simulink model "ALU_04_SS"  (R2022a)
settings: Solver=VariableStepAuto  StartTime=0.0  StopTime=10.0  RelTol=1e-3
undefined symbols (not defined in the file or in its folder): xc7z010iclg225
libraries: hdlBasic x1537, vmcUtilities x1
(part 8 of 8)

== system ALU_04_SS/ALU_64_BITS/ALU_63 ==
  CARRY_IN (1 BIT) : Inport
  OP (2 BIT) : Inport  Port=2
  A_INVERT (1 BIT) : Inport  Port=3
  A_INPUT (1 BIT) : Inport  Port=4
  B_INVERT (1 BIT) : Inport  Port=5
  B_INPUT (1 BIT) : Inport  Port=6
  Inverter{1..3,8..9} (5 alike) : hdlBasic/Inverter  en=off  latency=0  XmcBlockStatus=1  maskContainerNames=group2  block_type=inv  block_config=sysgen:Inverter_config
  Logical{,1..3} (4 alike) : hdlBasic/Logical  logical_function=AND  inputs=2  en=off  latency=0  precision=Full  arith_type=Unsigned  n_bits=16  bin_pt=0  align_bp=on  overflow=[]  quantization=[]  XmcBlockStatus=1  maskContainerNames=tabcontainer1  block_type=logical  block_config=sysgen:Logical_config
  Logical{4..6,9} (4 alike) : hdlBasic/Logical  logical_function=AND  inputs=3  en=off  latency=0  precision=Full  arith_type=Unsigned  n_bits=16  bin_pt=0  align_bp=on  overflow=[]  quantization=[]  XmcBlockStatus=1  maskContainerNames=tabcontainer1  block_type=logical  block_config=sysgen:Logical_config
  Logical7 : hdlBasic/Logical  logical_function=OR  inputs=2  en=off  latency=0  precision=Full  arith_type=Unsigned  n_bits=16  bin_pt=0  align_bp=on  overflow=[]  quantization=[]  XmcBlockStatus=1  maskContainerNames=tabcontainer1  block_type=logical  block_config=sysgen:Logical_config
  Logical8 : hdlBasic/Logical  logical_function=XOR  inputs=2  en=off  latency=0  precision=Full  arith_type=Unsigned  n_bits=16  bin_pt=0  align_bp=on  overflow=[]  quantization=[]  XmcBlockStatus=1  maskContainerNames=tabcontainer1  block_type=logical  block_config=sysgen:Logical_config
  Mux : hdlBasic/Mux  inputs=4  en=off  latency=0  precision=Full  arith_type=Unsigned  n_bits=16  bin_pt=14  quantization=Truncate  overflow=Wrap  XmcBlockStatus=1  maskContainerNames=tabcontainer1  block_type=mux  block_config=sysgen:Mux_config
  Mux1 : hdlBasic/Mux  inputs=2  en=off  latency=0  precision=Full  arith_type=Unsigned  n_bits=16  bin_pt=14  quantization=Truncate  overflow=Wrap  XmcBlockStatus=1  maskContainerNames=tabcontainer1  block_type=mux  block_config=sysgen:Mux_config
  Mux2 : hdlBasic/Mux  inputs=2  en=off  latency=0  precision=Full  arith_type=Unsigned  n_bits=16  bin_pt=14  quantization=Truncate  overflow=Wrap  XmcBlockStatus=1  maskContainerNames=tabcontainer1  block_type=mux  block_config=sysgen:Mux_config
  Sum : hdlBasic/Logical  logical_function=OR  inputs=4  en=off  latency=0  precision=Full  arith_type=Unsigned  n_bits=16  bin_pt=0  align_bp=on  overflow=[]  quantization=[]  XmcBlockStatus=1  maskContainerNames=tabcontainer1  block_type=logical  block_config=sysgen:Logical_config
  c_out : hdlBasic/Logical  logical_function=OR  inputs=3  en=off  latency=0  precision=Full  arith_type=Unsigned  n_bits=16  bin_pt=0  align_bp=on  overflow=[]  quantization=[]  XmcBlockStatus=1  maskContainerNames=tabcontainer1  block_type=logical  block_config=sysgen:Logical_config
  ALU_OUT (1 BIT) : Outport
  CARRY_OUT (1 BIT) : Outport  Port=2
  wires:
  Logical2/1 -> c_out/3
  A_INVERT (1 BIT)/1 -> Mux1/1
  c_out/1 -> CARRY_OUT (1 BIT)/1
  Sum/1 -> Mux/4
  CARRY_IN (1 BIT)/1 -> Inverter1/1, Logical5/1, Logical4/1, Logical1/1, Logical/1
  Mux2/1 -> Logical5/3, Logical6/3, Logical1/2, Logical2/2, Inverter9/1, Logical8/2, Logical3/2, Logical7/2
  B_INPUT (1 BIT)/1 -> Inverter3/1, Mux2/2
  Mux/1 -> ALU_OUT (1 BIT)/1
  Logical/1 -> c_out/1
  B_INVERT (1 BIT)/1 -> Mux2/1
  Logical6/1 -> Sum/3
  Mux1/1 -> Logical8/1, Logical7/1, Logical3/1, Inverter8/1, Logical5/2, Logical/2, Logical2/1, Logical9/2
  Logical5/1 -> Sum/4
  OP (2 BIT)/1 -> Mux/1
  Logical9/1 -> Sum/2
  Inverter1/1 -> Logical6/1, Logical9/1
  Inverter3/1 -> Mux2/3
  Inverter9/1 -> Logical9/3, Logical4/3
  A_INPUT (1 BIT)/1 -> Mux1/2, Inverter2/1
  Inverter2/1 -> Mux1/3
  Logical4/1 -> Sum/1
  Inverter8/1 -> Logical6/2, Logical4/2
  Logical3/1 -> Mux/2
  Logical7/1 -> Mux/3
  Logical1/1 -> c_out/2
  Logical8/1 -> Mux/5

== system ALU_04_SS/ALU_64_BITS/ALU_7 ==
  CARRY_IN (1 BIT) : Inport
  OP (2 BIT) : Inport  Port=2
  A_INVERT (1 BIT) : Inport  Port=3
  A_INPUT (1 BIT) : Inport  Port=4
  B_INVERT (1 BIT) : Inport  Port=5
  B_INPUT (1 BIT) : Inport  Port=6
  Inverter{1..3,8..9} (5 alike) : hdlBasic/Inverter  en=off  latency=0  XmcBlockStatus=1  maskContainerNames=group2  block_type=inv  block_config=sysgen:Inverter_config
  Logical{,1..3} (4 alike) : hdlBasic/Logical  logical_function=AND  inputs=2  en=off  latency=0  precision=Full  arith_type=Unsigned  n_bits=16  bin_pt=0  align_bp=on  overflow=[]  quantization=[]  XmcBlockStatus=1  maskContainerNames=tabcontainer1  block_type=logical  block_config=sysgen:Logical_config
  Logical{4..6,9} (4 alike) : hdlBasic/Logical  logical_function=AND  inputs=3  en=off  latency=0  precision=Full  arith_type=Unsigned  n_bits=16  bin_pt=0  align_bp=on  overflow=[]  quantization=[]  XmcBlockStatus=1  maskContainerNames=tabcontainer1  block_type=logical  block_config=sysgen:Logical_config
  Logical7 : hdlBasic/Logical  logical_function=OR  inputs=2  en=off  latency=0  precision=Full  arith_type=Unsigned  n_bits=16  bin_pt=0  align_bp=on  overflow=[]  quantization=[]  XmcBlockStatus=1  maskContainerNames=tabcontainer1  block_type=logical  block_config=sysgen:Logical_config
  Logical8 : hdlBasic/Logical  logical_function=XOR  inputs=2  en=off  latency=0  precision=Full  arith_type=Unsigned  n_bits=16  bin_pt=0  align_bp=on  overflow=[]  quantization=[]  XmcBlockStatus=1  maskContainerNames=tabcontainer1  block_type=logical  block_config=sysgen:Logical_config
  Mux : hdlBasic/Mux  inputs=4  en=off  latency=0  precision=Full  arith_type=Unsigned  n_bits=16  bin_pt=14  quantization=Truncate  overflow=Wrap  XmcBlockStatus=1  maskContainerNames=tabcontainer1  block_type=mux  block_config=sysgen:Mux_config
  Mux1 : hdlBasic/Mux  inputs=2  en=off  latency=0  precision=Full  arith_type=Unsigned  n_bits=16  bin_pt=14  quantization=Truncate  overflow=Wrap  XmcBlockStatus=1  maskContainerNames=tabcontainer1  block_type=mux  block_config=sysgen:Mux_config
  Mux2 : hdlBasic/Mux  inputs=2  en=off  latency=0  precision=Full  arith_type=Unsigned  n_bits=16  bin_pt=14  quantization=Truncate  overflow=Wrap  XmcBlockStatus=1  maskContainerNames=tabcontainer1  block_type=mux  block_config=sysgen:Mux_config
  Sum : hdlBasic/Logical  logical_function=OR  inputs=4  en=off  latency=0  precision=Full  arith_type=Unsigned  n_bits=16  bin_pt=0  align_bp=on  overflow=[]  quantization=[]  XmcBlockStatus=1  maskContainerNames=tabcontainer1  block_type=logical  block_config=sysgen:Logical_config
  c_out : hdlBasic/Logical  logical_function=OR  inputs=3  en=off  latency=0  precision=Full  arith_type=Unsigned  n_bits=16  bin_pt=0  align_bp=on  overflow=[]  quantization=[]  XmcBlockStatus=1  maskContainerNames=tabcontainer1  block_type=logical  block_config=sysgen:Logical_config
  ALU_OUT (1 BIT) : Outport
  CARRY_OUT (1 BIT) : Outport  Port=2
  wires:
  Logical2/1 -> c_out/3
  A_INVERT (1 BIT)/1 -> Mux1/1
  c_out/1 -> CARRY_OUT (1 BIT)/1
  Sum/1 -> Mux/4
  CARRY_IN (1 BIT)/1 -> Inverter1/1, Logical5/1, Logical4/1, Logical1/1, Logical/1
  Mux2/1 -> Logical5/3, Logical6/3, Logical1/2, Logical2/2, Inverter9/1, Logical8/2, Logical3/2, Logical7/2
  B_INPUT (1 BIT)/1 -> Inverter3/1, Mux2/2
  Mux/1 -> ALU_OUT (1 BIT)/1
  Logical/1 -> c_out/1
  B_INVERT (1 BIT)/1 -> Mux2/1
  Logical6/1 -> Sum/3
  Mux1/1 -> Logical8/1, Logical7/1, Logical3/1, Inverter8/1, Logical5/2, Logical/2, Logical2/1, Logical9/2
  Logical5/1 -> Sum/4
  OP (2 BIT)/1 -> Mux/1
  Logical9/1 -> Sum/2
  Inverter1/1 -> Logical6/1, Logical9/1
  Inverter3/1 -> Mux2/3
  Inverter9/1 -> Logical9/3, Logical4/3
  A_INPUT (1 BIT)/1 -> Mux1/2, Inverter2/1
  Inverter2/1 -> Mux1/3
  Logical4/1 -> Sum/1
  Inverter8/1 -> Logical6/2, Logical4/2
  Logical3/1 -> Mux/2
  Logical7/1 -> Mux/3
  Logical1/1 -> c_out/2
  Logical8/1 -> Mux/5

== system ALU_04_SS/ALU_64_BITS/ALU_8 ==
  CARRY_IN (1 BIT) : Inport
  OP (2 BIT) : Inport  Port=2
  A_INVERT (1 BIT) : Inport  Port=3
  A_INPUT (1 BIT) : Inport  Port=4
  B_INVERT (1 BIT) : Inport  Port=5
  B_INPUT (1 BIT) : Inport  Port=6
  Inverter{1..3,8..9} (5 alike) : hdlBasic/Inverter  en=off  latency=0  XmcBlockStatus=1  maskContainerNames=group2  block_type=inv  block_config=sysgen:Inverter_config
  Logical{,1..3} (4 alike) : hdlBasic/Logical  logical_function=AND  inputs=2  en=off  latency=0  precision=Full  arith_type=Unsigned  n_bits=16  bin_pt=0  align_bp=on  overflow=[]  quantization=[]  XmcBlockStatus=1  maskContainerNames=tabcontainer1  block_type=logical  block_config=sysgen:Logical_config
  Logical{4..6,9} (4 alike) : hdlBasic/Logical  logical_function=AND  inputs=3  en=off  latency=0  precision=Full  arith_type=Unsigned  n_bits=16  bin_pt=0  align_bp=on  overflow=[]  quantization=[]  XmcBlockStatus=1  maskContainerNames=tabcontainer1  block_type=logical  block_config=sysgen:Logical_config
  Logical7 : hdlBasic/Logical  logical_function=OR  inputs=2  en=off  latency=0  precision=Full  arith_type=Unsigned  n_bits=16  bin_pt=0  align_bp=on  overflow=[]  quantization=[]  XmcBlockStatus=1  maskContainerNames=tabcontainer1  block_type=logical  block_config=sysgen:Logical_config
  Logical8 : hdlBasic/Logical  logical_function=XOR  inputs=2  en=off  latency=0  precision=Full  arith_type=Unsigned  n_bits=16  bin_pt=0  align_bp=on  overflow=[]  quantization=[]  XmcBlockStatus=1  maskContainerNames=tabcontainer1  block_type=logical  block_config=sysgen:Logical_config
  Mux : hdlBasic/Mux  inputs=4  en=off  latency=0  precision=Full  arith_type=Unsigned  n_bits=16  bin_pt=14  quantization=Truncate  overflow=Wrap  XmcBlockStatus=1  maskContainerNames=tabcontainer1  block_type=mux  block_config=sysgen:Mux_config
  Mux1 : hdlBasic/Mux  inputs=2  en=off  latency=0  precision=Full  arith_type=Unsigned  n_bits=16  bin_pt=14  quantization=Truncate  overflow=Wrap  XmcBlockStatus=1  maskContainerNames=tabcontainer1  block_type=mux  block_config=sysgen:Mux_config
  Mux2 : hdlBasic/Mux  inputs=2  en=off  latency=0  precision=Full  arith_type=Unsigned  n_bits=16  bin_pt=14  quantization=Truncate  overflow=Wrap  XmcBlockStatus=1  maskContainerNames=tabcontainer1  block_type=mux  block_config=sysgen:Mux_config
  Sum : hdlBasic/Logical  logical_function=OR  inputs=4  en=off  latency=0  precision=Full  arith_type=Unsigned  n_bits=16  bin_pt=0  align_bp=on  overflow=[]  quantization=[]  XmcBlockStatus=1  maskContainerNames=tabcontainer1  block_type=logical  block_config=sysgen:Logical_config
  c_out : hdlBasic/Logical  logical_function=OR  inputs=3  en=off  latency=0  precision=Full  arith_type=Unsigned  n_bits=16  bin_pt=0  align_bp=on  overflow=[]  quantization=[]  XmcBlockStatus=1  maskContainerNames=tabcontainer1  block_type=logical  block_config=sysgen:Logical_config
  ALU_OUT (1 BIT) : Outport
  CARRY_OUT (1 BIT) : Outport  Port=2
  wires:
  Logical2/1 -> c_out/3
  A_INVERT (1 BIT)/1 -> Mux1/1
  c_out/1 -> CARRY_OUT (1 BIT)/1
  Sum/1 -> Mux/4
  CARRY_IN (1 BIT)/1 -> Inverter1/1, Logical5/1, Logical4/1, Logical1/1, Logical/1
  Mux2/1 -> Logical5/3, Logical6/3, Logical1/2, Logical2/2, Inverter9/1, Logical8/2, Logical3/2, Logical7/2
  B_INPUT (1 BIT)/1 -> Inverter3/1, Mux2/2
  Mux/1 -> ALU_OUT (1 BIT)/1
  Logical/1 -> c_out/1
  B_INVERT (1 BIT)/1 -> Mux2/1
  Logical6/1 -> Sum/3
  Mux1/1 -> Logical8/1, Logical7/1, Logical3/1, Inverter8/1, Logical5/2, Logical/2, Logical2/1, Logical9/2
  Logical5/1 -> Sum/4
  OP (2 BIT)/1 -> Mux/1
  Logical9/1 -> Sum/2
  Inverter1/1 -> Logical6/1, Logical9/1
  Inverter3/1 -> Mux2/3
  Inverter9/1 -> Logical9/3, Logical4/3
  A_INPUT (1 BIT)/1 -> Mux1/2, Inverter2/1
  Inverter2/1 -> Mux1/3
  Logical4/1 -> Sum/1
  Inverter8/1 -> Logical6/2, Logical4/2
  Logical3/1 -> Mux/2
  Logical7/1 -> Mux/3
  Logical1/1 -> c_out/2
  Logical8/1 -> Mux/5

== system ALU_04_SS/ALU_64_BITS/ALU_9 ==
  CARRY_IN (1 BIT) : Inport
  OP (2 BIT) : Inport  Port=2
  A_INVERT (1 BIT) : Inport  Port=3
  A_INPUT (1 BIT) : Inport  Port=4
  B_INVERT (1 BIT) : Inport  Port=5
  B_INPUT (1 BIT) : Inport  Port=6
  Inverter{1..3,8..9} (5 alike) : hdlBasic/Inverter  en=off  latency=0  XmcBlockStatus=1  maskContainerNames=group2  block_type=inv  block_config=sysgen:Inverter_config
  Logical{,1..3} (4 alike) : hdlBasic/Logical  logical_function=AND  inputs=2  en=off  latency=0  precision=Full  arith_type=Unsigned  n_bits=16  bin_pt=0  align_bp=on  overflow=[]  quantization=[]  XmcBlockStatus=1  maskContainerNames=tabcontainer1  block_type=logical  block_config=sysgen:Logical_config
  Logical{4..6,9} (4 alike) : hdlBasic/Logical  logical_function=AND  inputs=3  en=off  latency=0  precision=Full  arith_type=Unsigned  n_bits=16  bin_pt=0  align_bp=on  overflow=[]  quantization=[]  XmcBlockStatus=1  maskContainerNames=tabcontainer1  block_type=logical  block_config=sysgen:Logical_config
  Logical7 : hdlBasic/Logical  logical_function=OR  inputs=2  en=off  latency=0  precision=Full  arith_type=Unsigned  n_bits=16  bin_pt=0  align_bp=on  overflow=[]  quantization=[]  XmcBlockStatus=1  maskContainerNames=tabcontainer1  block_type=logical  block_config=sysgen:Logical_config
  Logical8 : hdlBasic/Logical  logical_function=XOR  inputs=2  en=off  latency=0  precision=Full  arith_type=Unsigned  n_bits=16  bin_pt=0  align_bp=on  overflow=[]  quantization=[]  XmcBlockStatus=1  maskContainerNames=tabcontainer1  block_type=logical  block_config=sysgen:Logical_config
  Mux : hdlBasic/Mux  inputs=4  en=off  latency=0  precision=Full  arith_type=Unsigned  n_bits=16  bin_pt=14  quantization=Truncate  overflow=Wrap  XmcBlockStatus=1  maskContainerNames=tabcontainer1  block_type=mux  block_config=sysgen:Mux_config
  Mux1 : hdlBasic/Mux  inputs=2  en=off  latency=0  precision=Full  arith_type=Unsigned  n_bits=16  bin_pt=14  quantization=Truncate  overflow=Wrap  XmcBlockStatus=1  maskContainerNames=tabcontainer1  block_type=mux  block_config=sysgen:Mux_config
  Mux2 : hdlBasic/Mux  inputs=2  en=off  latency=0  precision=Full  arith_type=Unsigned  n_bits=16  bin_pt=14  quantization=Truncate  overflow=Wrap  XmcBlockStatus=1  maskContainerNames=tabcontainer1  block_type=mux  block_config=sysgen:Mux_config
  Sum : hdlBasic/Logical  logical_function=OR  inputs=4  en=off  latency=0  precision=Full  arith_type=Unsigned  n_bits=16  bin_pt=0  align_bp=on  overflow=[]  quantization=[]  XmcBlockStatus=1  maskContainerNames=tabcontainer1  block_type=logical  block_config=sysgen:Logical_config
  c_out : hdlBasic/Logical  logical_function=OR  inputs=3  en=off  latency=0  precision=Full  arith_type=Unsigned  n_bits=16  bin_pt=0  align_bp=on  overflow=[]  quantization=[]  XmcBlockStatus=1  maskContainerNames=tabcontainer1  block_type=logical  block_config=sysgen:Logical_config
  ALU_OUT (1 BIT) : Outport
  CARRY_OUT (1 BIT) : Outport  Port=2
  wires:
  Logical2/1 -> c_out/3
  A_INVERT (1 BIT)/1 -> Mux1/1
  c_out/1 -> CARRY_OUT (1 BIT)/1
  Sum/1 -> Mux/4
  CARRY_IN (1 BIT)/1 -> Inverter1/1, Logical5/1, Logical4/1, Logical1/1, Logical/1
  Mux2/1 -> Logical5/3, Logical6/3, Logical1/2, Logical2/2, Inverter9/1, Logical8/2, Logical3/2, Logical7/2
  B_INPUT (1 BIT)/1 -> Inverter3/1, Mux2/2
  Mux/1 -> ALU_OUT (1 BIT)/1
  Logical/1 -> c_out/1
  B_INVERT (1 BIT)/1 -> Mux2/1
  Logical6/1 -> Sum/3
  Mux1/1 -> Logical8/1, Logical7/1, Logical3/1, Inverter8/1, Logical5/2, Logical/2, Logical2/1, Logical9/2
  Logical5/1 -> Sum/4
  OP (2 BIT)/1 -> Mux/1
  Logical9/1 -> Sum/2
  Inverter1/1 -> Logical6/1, Logical9/1
  Inverter3/1 -> Mux2/3
  Inverter9/1 -> Logical9/3, Logical4/3
  A_INPUT (1 BIT)/1 -> Mux1/2, Inverter2/1
  Inverter2/1 -> Mux1/3
  Logical4/1 -> Sum/1
  Inverter8/1 -> Logical6/2, Logical4/2
  Logical3/1 -> Mux/2
  Logical7/1 -> Mux/3
  Logical1/1 -> c_out/2
  Logical8/1 -> Mux/5

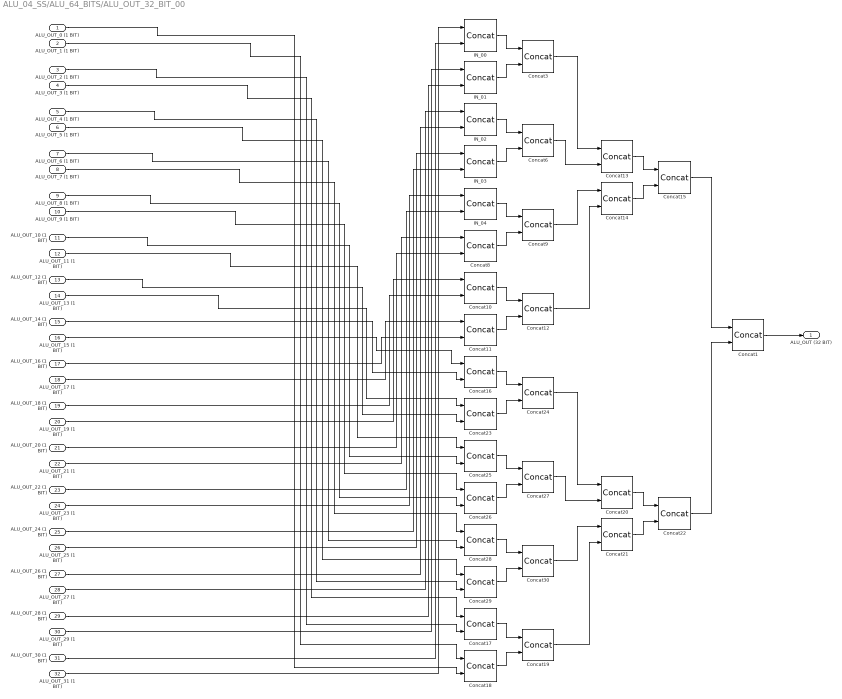
== system ALU_04_SS/ALU_64_BITS/ALU_OUT_32_BIT_00 ==
  ALU_OUT_0 (1 BIT) : Inport
  ALU_OUT_1 (1 BIT) : Inport  Port=2
  ALU_OUT_2 (1 BIT) : Inport  Port=3
  ALU_OUT_3 (1 BIT) : Inport  Port=4
  ALU_OUT_4 (1 BIT) : Inport  Port=5
  ALU_OUT_5 (1 BIT) : Inport  Port=6
  ALU_OUT_6 (1 BIT) : Inport  Port=7
  ALU_OUT_7 (1 BIT) : Inport  Port=8
  ALU_OUT_8 (1 BIT) : Inport  Port=9
  ALU_OUT_9 (1 BIT) : Inport  Port=10
  ALU_OUT_10 (1 BIT) : Inport  Port=11
  ALU_OUT_11 (1 BIT) : Inport  Port=12
  ALU_OUT_12 (1 BIT) : Inport  Port=13
  ALU_OUT_13 (1 BIT) : Inport  Port=14
  ALU_OUT_14 (1 BIT) : Inport  Port=15
  ALU_OUT_15 (1 BIT) : Inport  Port=16
  ALU_OUT_16 (1 BIT) : Inport  Port=17
  ALU_OUT_17 (1 BIT) : Inport  Port=18
  ALU_OUT_18 (1 BIT) : Inport  Port=19
  ALU_OUT_19 (1 BIT) : Inport  Port=20
  ALU_OUT_20 (1 BIT) : Inport  Port=21
  ALU_OUT_21 (1 BIT) : Inport  Port=22
  ALU_OUT_22 (1 BIT) : Inport  Port=23
  ALU_OUT_23 (1 BIT) : Inport  Port=24
  ALU_OUT_24 (1 BIT) : Inport  Port=25
  ALU_OUT_25 (1 BIT) : Inport  Port=26
  ALU_OUT_26 (1 BIT) : Inport  Port=27
  ALU_OUT_27 (1 BIT) : Inport  Port=28
  ALU_OUT_28 (1 BIT) : Inport  Port=29
  ALU_OUT_29 (1 BIT) : Inport  Port=30
  ALU_OUT_30 (1 BIT) : Inport  Port=31
  ALU_OUT_31 (1 BIT) : Inport  Port=32
  Concat{1,3,6,8..30} (26 alike) : hdlBasic/Concat  num_inputs=2  XmcBlockStatus=1  maskContainerNames=group1  block_type=concat  block_config=sysgen:Concat_config
  IN_00 : hdlBasic/Concat  num_inputs=2  XmcBlockStatus=1  maskContainerNames=group1  block_type=concat  block_config=sysgen:Concat_config
  IN_01 : hdlBasic/Concat  num_inputs=2  XmcBlockStatus=1  maskContainerNames=group1  block_type=concat  block_config=sysgen:Concat_config
  IN_02 : hdlBasic/Concat  num_inputs=2  XmcBlockStatus=1  maskContainerNames=group1  block_type=concat  block_config=sysgen:Concat_config
  IN_03 : hdlBasic/Concat  num_inputs=2  XmcBlockStatus=1  maskContainerNames=group1  block_type=concat  block_config=sysgen:Concat_config
  IN_04 : hdlBasic/Concat  num_inputs=2  XmcBlockStatus=1  maskContainerNames=group1  block_type=concat  block_config=sysgen:Concat_config
  ALU_OUT (32 BIT) : Outport
  wires:
  IN_01/1 -> Concat3/2
  Concat10/1 -> Concat12/1
  Concat27/1 -> Concat20/2
  Concat19/1 -> Concat21/2
  Concat22/1 -> Concat1/2
  Concat28/1 -> Concat30/1
  Concat11/1 -> Concat12/2
  Concat29/1 -> Concat30/2
  Concat21/1 -> Concat22/2
  IN_00/1 -> Concat3/1
  Concat3/1 -> Concat13/1
  Concat20/1 -> Concat22/1
  Concat17/1 -> Concat19/1
  Concat26/1 -> Concat27/2
  Concat6/1 -> Concat13/2
  Concat13/1 -> Concat15/1
  Concat30/1 -> Concat21/1
  Concat24/1 -> Concat20/1
  Concat16/1 -> Concat24/1
  Concat23/1 -> Concat24/2
  Concat18/1 -> Concat19/2
  Concat25/1 -> Concat27/1
  IN_02/1 -> Concat6/1
  IN_03/1 -> Concat6/2
  Concat9/1 -> Concat14/1
  Concat15/1 -> Concat1/1
  Concat8/1 -> Concat9/2
  IN_04/1 -> Concat9/1
  Concat14/1 -> Concat15/2
  Concat12/1 -> Concat14/2
  Concat1/1 -> ALU_OUT (32 BIT)/1
  ALU_OUT_31 (1 BIT)/1 -> IN_00/1
  ALU_OUT_30 (1 BIT)/1 -> IN_00/2
  ALU_OUT_29 (1 BIT)/1 -> IN_01/1
  ALU_OUT_28 (1 BIT)/1 -> IN_01/2
  ALU_OUT_27 (1 BIT)/1 -> IN_02/1
  ALU_OUT_26 (1 BIT)/1 -> IN_02/2
  ALU_OUT_25 (1 BIT)/1 -> IN_03/1
  ALU_OUT_24 (1 BIT)/1 -> IN_03/2
  ALU_OUT_23 (1 BIT)/1 -> IN_04/1
  ALU_OUT_22 (1 BIT)/1 -> IN_04/2
  ALU_OUT_21 (1 BIT)/1 -> Concat8/1
  ALU_OUT_20 (1 BIT)/1 -> Concat8/2
  ALU_OUT_19 (1 BIT)/1 -> Concat10/1
  ALU_OUT_18 (1 BIT)/1 -> Concat10/2
  ALU_OUT_17 (1 BIT)/1 -> Concat11/1
  ALU_OUT_16 (1 BIT)/1 -> Concat11/2
  ALU_OUT_15 (1 BIT)/1 -> Concat16/1
  ALU_OUT_14 (1 BIT)/1 -> Concat16/2
  ALU_OUT_13 (1 BIT)/1 -> Concat23/1
  ALU_OUT_12 (1 BIT)/1 -> Concat23/2
  ALU_OUT_11 (1 BIT)/1 -> Concat25/1
  ALU_OUT_10 (1 BIT)/1 -> Concat25/2
  ALU_OUT_9 (1 BIT)/1 -> Concat26/1
  ALU_OUT_8 (1 BIT)/1 -> Concat26/2
  ALU_OUT_7 (1 BIT)/1 -> Concat28/1
  ALU_OUT_6 (1 BIT)/1 -> Concat28/2
  ALU_OUT_5 (1 BIT)/1 -> Concat29/1
  ALU_OUT_4 (1 BIT)/1 -> Concat29/2
  ALU_OUT_3 (1 BIT)/1 -> Concat17/1
  ALU_OUT_2 (1 BIT)/1 -> Concat17/2
  ALU_OUT_1 (1 BIT)/1 -> Concat18/1
  ALU_OUT_0 (1 BIT)/1 -> Concat18/2

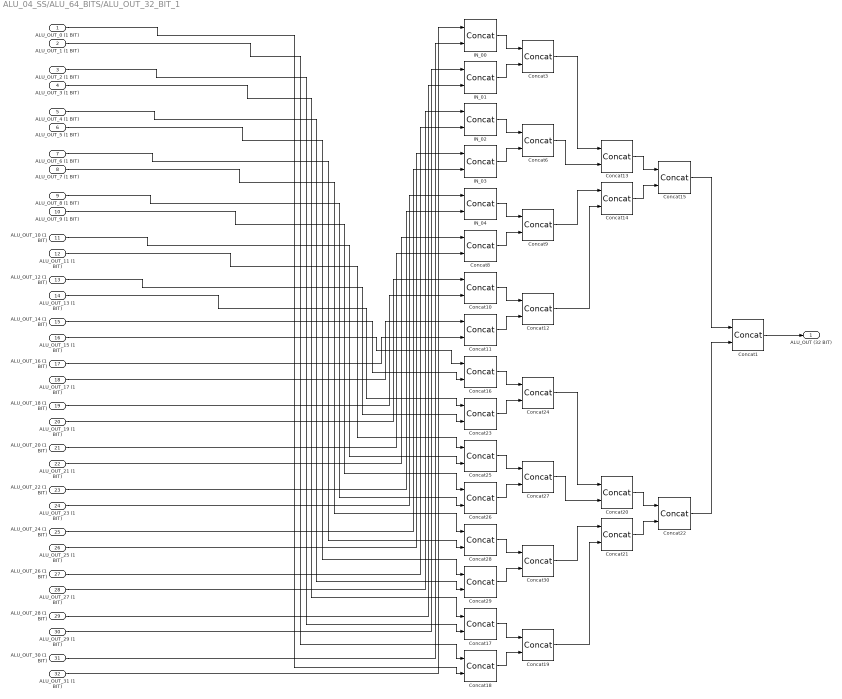
== system ALU_04_SS/ALU_64_BITS/ALU_OUT_32_BIT_1 ==
  ALU_OUT_0 (1 BIT) : Inport
  ALU_OUT_1 (1 BIT) : Inport  Port=2
  ALU_OUT_2 (1 BIT) : Inport  Port=3
  ALU_OUT_3 (1 BIT) : Inport  Port=4
  ALU_OUT_4 (1 BIT) : Inport  Port=5
  ALU_OUT_5 (1 BIT) : Inport  Port=6
  ALU_OUT_6 (1 BIT) : Inport  Port=7
  ALU_OUT_7 (1 BIT) : Inport  Port=8
  ALU_OUT_8 (1 BIT) : Inport  Port=9
  ALU_OUT_9 (1 BIT) : Inport  Port=10
  ALU_OUT_10 (1 BIT) : Inport  Port=11
  ALU_OUT_11 (1 BIT) : Inport  Port=12
  ALU_OUT_12 (1 BIT) : Inport  Port=13
  ALU_OUT_13 (1 BIT) : Inport  Port=14
  ALU_OUT_14 (1 BIT) : Inport  Port=15
  ALU_OUT_15 (1 BIT) : Inport  Port=16
  ALU_OUT_16 (1 BIT) : Inport  Port=17
  ALU_OUT_17 (1 BIT) : Inport  Port=18
  ALU_OUT_18 (1 BIT) : Inport  Port=19
  ALU_OUT_19 (1 BIT) : Inport  Port=20
  ALU_OUT_20 (1 BIT) : Inport  Port=21
  ALU_OUT_21 (1 BIT) : Inport  Port=22
  ALU_OUT_22 (1 BIT) : Inport  Port=23
  ALU_OUT_23 (1 BIT) : Inport  Port=24
  ALU_OUT_24 (1 BIT) : Inport  Port=25
  ALU_OUT_25 (1 BIT) : Inport  Port=26
  ALU_OUT_26 (1 BIT) : Inport  Port=27
  ALU_OUT_27 (1 BIT) : Inport  Port=28
  ALU_OUT_28 (1 BIT) : Inport  Port=29
  ALU_OUT_29 (1 BIT) : Inport  Port=30
  ALU_OUT_30 (1 BIT) : Inport  Port=31
  ALU_OUT_31 (1 BIT) : Inport  Port=32
  Concat{1,3,6,8..30} (26 alike) : hdlBasic/Concat  num_inputs=2  XmcBlockStatus=1  maskContainerNames=group1  block_type=concat  block_config=sysgen:Concat_config
  IN_00 : hdlBasic/Concat  num_inputs=2  XmcBlockStatus=1  maskContainerNames=group1  block_type=concat  block_config=sysgen:Concat_config
  IN_01 : hdlBasic/Concat  num_inputs=2  XmcBlockStatus=1  maskContainerNames=group1  block_type=concat  block_config=sysgen:Concat_config
  IN_02 : hdlBasic/Concat  num_inputs=2  XmcBlockStatus=1  maskContainerNames=group1  block_type=concat  block_config=sysgen:Concat_config
  IN_03 : hdlBasic/Concat  num_inputs=2  XmcBlockStatus=1  maskContainerNames=group1  block_type=concat  block_config=sysgen:Concat_config
  IN_04 : hdlBasic/Concat  num_inputs=2  XmcBlockStatus=1  maskContainerNames=group1  block_type=concat  block_config=sysgen:Concat_config
  ALU_OUT (32 BIT) : Outport
  wires:
  IN_01/1 -> Concat3/2
  Concat10/1 -> Concat12/1
  Concat27/1 -> Concat20/2
  Concat19/1 -> Concat21/2
  Concat22/1 -> Concat1/2
  Concat28/1 -> Concat30/1
  Concat11/1 -> Concat12/2
  Concat29/1 -> Concat30/2
  Concat21/1 -> Concat22/2
  IN_00/1 -> Concat3/1
  Concat3/1 -> Concat13/1
  Concat20/1 -> Concat22/1
  Concat17/1 -> Concat19/1
  Concat26/1 -> Concat27/2
  Concat6/1 -> Concat13/2
  Concat13/1 -> Concat15/1
  Concat30/1 -> Concat21/1
  Concat24/1 -> Concat20/1
  Concat16/1 -> Concat24/1
  Concat23/1 -> Concat24/2
  Concat18/1 -> Concat19/2
  Concat25/1 -> Concat27/1
  IN_02/1 -> Concat6/1
  IN_03/1 -> Concat6/2
  Concat9/1 -> Concat14/1
  Concat15/1 -> Concat1/1
  Concat8/1 -> Concat9/2
  IN_04/1 -> Concat9/1
  Concat14/1 -> Concat15/2
  Concat12/1 -> Concat14/2
  Concat1/1 -> ALU_OUT (32 BIT)/1
  ALU_OUT_31 (1 BIT)/1 -> IN_00/1
  ALU_OUT_30 (1 BIT)/1 -> IN_00/2
  ALU_OUT_29 (1 BIT)/1 -> IN_01/1
  ALU_OUT_28 (1 BIT)/1 -> IN_01/2
  ALU_OUT_27 (1 BIT)/1 -> IN_02/1
  ALU_OUT_26 (1 BIT)/1 -> IN_02/2
  ALU_OUT_25 (1 BIT)/1 -> IN_03/1
  ALU_OUT_24 (1 BIT)/1 -> IN_03/2
  ALU_OUT_23 (1 BIT)/1 -> IN_04/1
  ALU_OUT_22 (1 BIT)/1 -> IN_04/2
  ALU_OUT_21 (1 BIT)/1 -> Concat8/1
  ALU_OUT_20 (1 BIT)/1 -> Concat8/2
  ALU_OUT_19 (1 BIT)/1 -> Concat10/1
  ALU_OUT_18 (1 BIT)/1 -> Concat10/2
  ALU_OUT_17 (1 BIT)/1 -> Concat11/1
  ALU_OUT_16 (1 BIT)/1 -> Concat11/2
  ALU_OUT_15 (1 BIT)/1 -> Concat16/1
  ALU_OUT_14 (1 BIT)/1 -> Concat16/2
  ALU_OUT_13 (1 BIT)/1 -> Concat23/1
  ALU_OUT_12 (1 BIT)/1 -> Concat23/2
  ALU_OUT_11 (1 BIT)/1 -> Concat25/1
  ALU_OUT_10 (1 BIT)/1 -> Concat25/2
  ALU_OUT_9 (1 BIT)/1 -> Concat26/1
  ALU_OUT_8 (1 BIT)/1 -> Concat26/2
  ALU_OUT_7 (1 BIT)/1 -> Concat28/1
  ALU_OUT_6 (1 BIT)/1 -> Concat28/2
  ALU_OUT_5 (1 BIT)/1 -> Concat29/1
  ALU_OUT_4 (1 BIT)/1 -> Concat29/2
  ALU_OUT_3 (1 BIT)/1 -> Concat17/1
  ALU_OUT_2 (1 BIT)/1 -> Concat17/2
  ALU_OUT_1 (1 BIT)/1 -> Concat18/1
  ALU_OUT_0 (1 BIT)/1 -> Concat18/2
